simulink model "ANC_simulation_all"  (R2023b)
settings: Solver=VariableStepAuto  StartTime=0.0  StopTime=1  RelTol=1e-3
model workspace (MAT data in the model file):
  A = 10
  Lp = 1
  Ls = 0.1
  Ts = 0.001
  c = 340
  f = 10
  step = 3
  x_product = 2
settings Model: Creator=nurbi  LastModifiedBy=nurbi

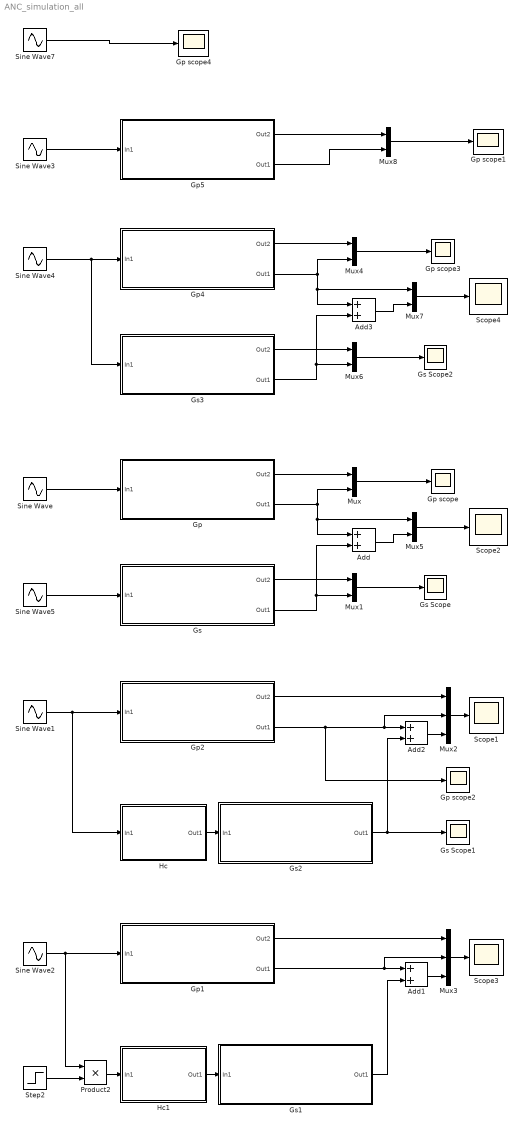
== system ANC_simulation_all ==
  Add{,1..3} (4 alike) : Sum
  Gp : Subsystem
  Gp scope{,1..4} (5 alike) : Scope
  Gp1 : Subsystem
  Gp2 : Subsystem
  Gp4 : Subsystem
  Gp5 : Subsystem
  Gs : Subsystem
  Gs Scope : Scope
  Gs Scope1 : Scope
  Gs Scope2 : Scope
  Gs1 : Subsystem
  Gs2 : Subsystem
  Gs3 : Subsystem
  Hc : Subsystem
  Hc1 : Subsystem
  Mux{,1,4..8} (7 alike) : Mux  Inputs=2
  Mux2 : Mux  Inputs=3
  Mux3 : Mux  Inputs=3
  Product2 : Product
  Scope{1..4} (4 alike) : Scope
  Sine Wave{,1..4} (5 alike) : Sin  Amplitude=A  Frequency=2*pi*f  SampleTime=0
  Sine Wave5 : Sin  Amplitude=5  Frequency=2*pi*f  SampleTime=0
  Sine Wave7 : Sin  Amplitude=A  Frequency=2*pi*f  SampleTime=Ts
  Step2 : Step  Time=0.5  SampleTime=0
  wires:
  Sine Wave/1 -> Gp/1(In1)
  Mux1/1 -> Gs Scope/1
  Gs/2(Out1) -> Mux1/2, Add/2
  Add/1 -> Mux5/2
  Gp/2(Out1) -> Add/1, Mux5/1, Mux/2
  Gs/1(Out2) -> Mux1/1
  Gp/1(Out2) -> Mux/1
  Mux5/1 -> Scope2/1
  Mux/1 -> Gp scope/1
  Gs2/1(Out1) -> Add2/2, Gs Scope1/1
  Hc/1(Out1) -> Gs2/1(In1)
  Sine Wave1/1 -> Hc/1(In1), Gp2/1(In1)
  Mux2/1 -> Scope1/1
  Add2/1 -> Mux2/3
  Sine Wave3/1 -> Gp5/1(In1)
  Gp2/2(Out1) -> Add2/1, Mux2/2, Gp scope2/1
  Gp2/1(Out2) -> Mux2/1
  Add1/1 -> Mux3/3
  Sine Wave2/1 -> Product2/1, Gp1/1(In1)
  Hc1/1(Out1) -> Gs1/1(In1)
  Step2/1 -> Product2/2
  Gs1/1(Out1) -> Add1/2
  Product2/1 -> Hc1/1(In1)
  Gp1/2(Out1) -> Mux3/2, Add1/1
  Mux3/1 -> Scope3/1
  Gp1/1(Out2) -> Mux3/1
  Gs3/2(Out1) -> Mux6/2, Add3/2
  Mux7/1 -> Scope4/1
  Mux4/1 -> Gp scope3/1
  Gp4/1(Out2) -> Mux4/1
  Mux6/1 -> Gs Scope2/1
  Sine Wave4/1 -> Gs3/1(In1), Gp4/1(In1)
  Gp4/2(Out1) -> Add3/1, Mux7/1, Mux4/2
  Add3/1 -> Mux7/2
  Gs3/1(Out2) -> Mux6/1
  Sine Wave5/1 -> Gs/1(In1)
  Gp5/1(Out2) -> Mux8/1
  Gp5/2(Out1) -> Mux8/2
  Mux8/1 -> Gp scope1/1
  Sine Wave7/1 -> Gp scope4/1

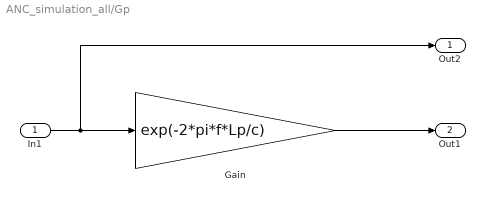
== system ANC_simulation_all/Gp ==
  In1 : Inport
  Gain : Gain  Gain=exp(-2*pi*f*Lp/c)
  Out2 : Outport
  Out1 : Outport  Port=2
  wires:
  In1/1 -> Out2/1, Gain/1
  Gain/1 -> Out1/1

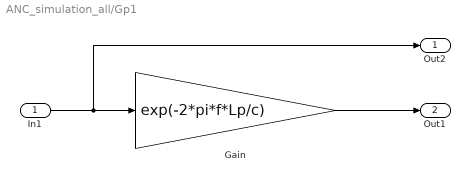
== system ANC_simulation_all/Gp1 ==
  In1 : Inport
  Gain : Gain  Gain=exp(-2*pi*f*Lp/c)
  Out2 : Outport
  Out1 : Outport  Port=2
  wires:
  In1/1 -> Gain/1, Out2/1
  Gain/1 -> Out1/1

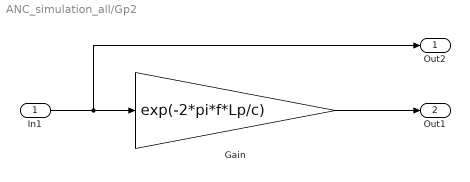
== system ANC_simulation_all/Gp2 ==
  In1 : Inport
  Gain : Gain  Gain=exp(-2*pi*f*Lp/c)
  Out2 : Outport
  Out1 : Outport  Port=2
  wires:
  In1/1 -> Gain/1, Out2/1
  Gain/1 -> Out1/1

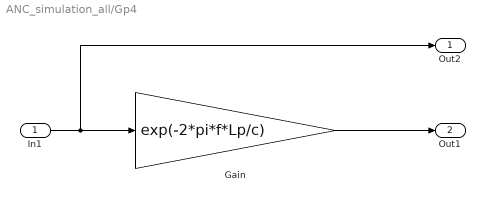
== system ANC_simulation_all/Gp4 ==
  In1 : Inport
  Gain : Gain  Gain=exp(-2*pi*f*Lp/c)
  Out2 : Outport
  Out1 : Outport  Port=2
  wires:
  In1/1 -> Out2/1, Gain/1
  Gain/1 -> Out1/1

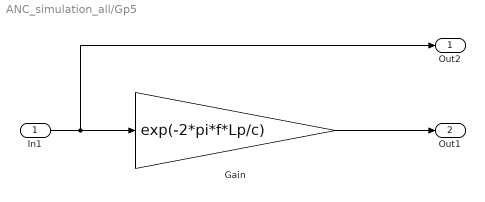
== system ANC_simulation_all/Gp5 ==
  In1 : Inport
  Gain : Gain  Gain=exp(-2*pi*f*Lp/c)
  Out2 : Outport
  Out1 : Outport  Port=2
  wires:
  In1/1 -> Out2/1, Gain/1
  Gain/1 -> Out1/1

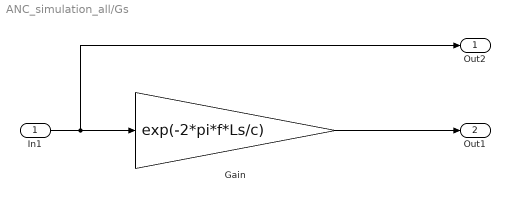
== system ANC_simulation_all/Gs ==
  In1 : Inport
  Gain : Gain  Gain=exp(-2*pi*f*Ls/c)
  Out2 : Outport
  Out1 : Outport  Port=2
  wires:
  In1/1 -> Out2/1, Gain/1
  Gain/1 -> Out1/1

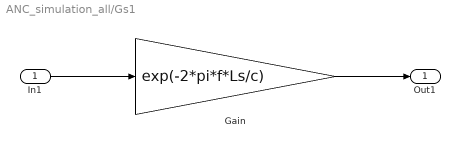
== system ANC_simulation_all/Gs1 ==
  In1 : Inport
  Gain : Gain  Gain=exp(-2*pi*f*Ls/c)
  Out1 : Outport
  wires:
  In1/1 -> Gain/1
  Gain/1 -> Out1/1

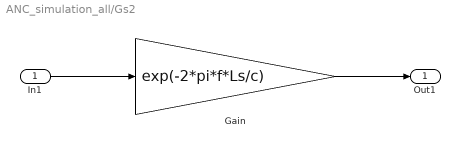
== system ANC_simulation_all/Gs2 ==
  In1 : Inport
  Gain : Gain  Gain=exp(-2*pi*f*Ls/c)
  Out1 : Outport
  wires:
  In1/1 -> Gain/1
  Gain/1 -> Out1/1

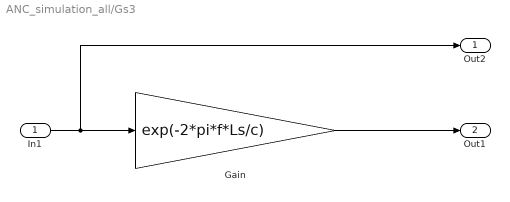
== system ANC_simulation_all/Gs3 ==
  In1 : Inport
  Gain : Gain  Gain=exp(-2*pi*f*Ls/c)
  Out2 : Outport
  Out1 : Outport  Port=2
  wires:
  In1/1 -> Out2/1, Gain/1
  Gain/1 -> Out1/1

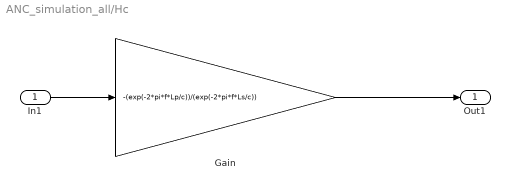
== system ANC_simulation_all/Hc ==
  In1 : Inport
  Gain : Gain  Gain=-(exp(-2*pi*f*Lp/c))/(exp(-2*pi*f*Ls/c))
  Out1 : Outport
  wires:
  Gain/1 -> Out1/1
  In1/1 -> Gain/1

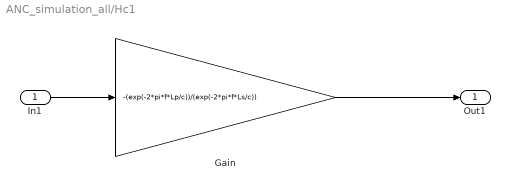
== system ANC_simulation_all/Hc1 ==
  In1 : Inport
  Gain : Gain  Gain=-(exp(-2*pi*f*Lp/c))/(exp(-2*pi*f*Ls/c))
  Out1 : Outport
  wires:
  Gain/1 -> Out1/1
  In1/1 -> Gain/1
